simulink model "adcddcxaui"  (Simulink 8.1)
settings: Solver=ode45  StartTime=0.0  StopTime=100  RelTol=1e-3
libraries: xbsIndex_r4 x407, xbsIndex_r3 x127, xps_library x29, casper_library x5, casper_library_misc x4, casper_library_scopes x3
(part 1 of 6)
settings Model: Creator=andrew  LastModifiedBy=andrew
settings OptimizationCC: ExpressionDepthLimit=128  InitFltsAndDblsToZero=on
settings DebuggingCC: SaveWithParameterizedLinksMsg=none  SignalResolutionControl=TryResolveAllWithWarning  MultiTaskDSMMsg=warning  MultiTaskCondExecSysMsg=none  StrictBusMsg=None
settings RTWCC: IncludeERTFirstTime=on
settings GRTTargetCC: TargetFcnLib=ansi_tfl_tmw.mat

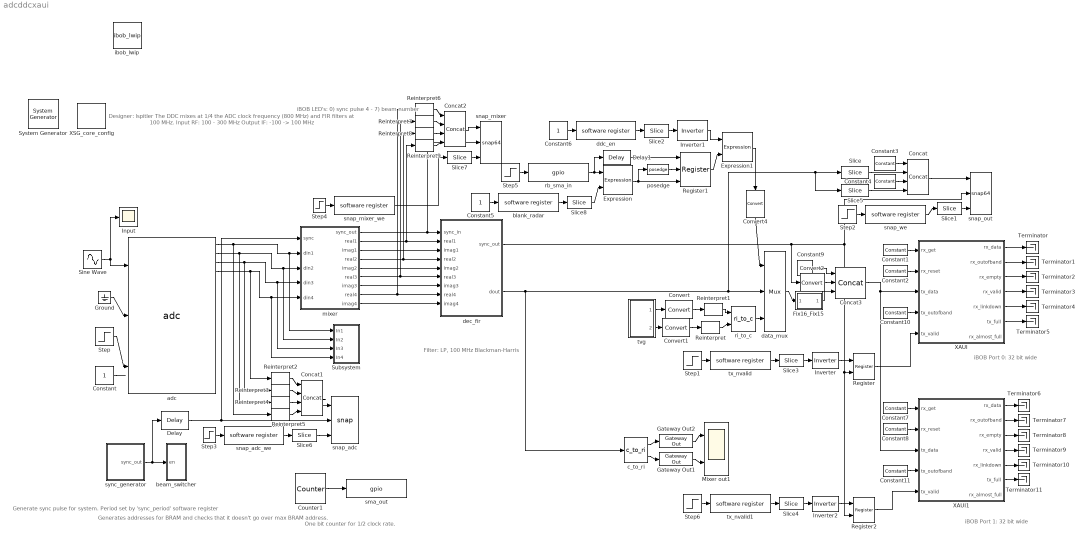
== system adcddcxaui ==
  note: Designer: lspitler
      | The DDC mixes at 1/4 the ADC clock frequency (800 MHz)
      | and FIR filters at 100 MHz.
      | Input RF: 100 - 300 MHz
      | Output IF: -100 -> 100 MHz
  note: Filter:
      | LP, 100 MHz Blackman-Harris
  note: iBOB Port 0: 32 bit wide
  note: One bit counter
      | for 1/2 clock rate.
  note: Generate sync pulse for system.
      | Period set by 'sync_period'
      | software register
  note: iBOB LED's:
      | 0) sync pulse
      | 4 - 7) beam number
  note: Generates addresses
      | for BRAM and checks
      | that it doesn't go over
      | max BRAM address.
  note: iBOB Port 1: 32 bit wide
  " System Generator" : xbsIndex_r4/ System Generator  Tag=genX  xilinxfamily=Kintex7  part=xc7k325t  speed=-3  package=fbg676  synthesis_tool=XST  clock_wrapper=Clock Enables  directory=./netlist  proj_type=Project Navigator  Synth_file=XST Defaults  Impl_file=ISE Defaults  testbench=off  simulink_period=1  sysclk_period=10  dcm_input_clock_period=10  incr_netlist=off  trim_vbits=Everywhere in SubSystem  dbl_ovrd=According to Block Masks  core_generation=According to Block Masks  run_coregen=off  deprecated_control=off  eval_field=0  block_type=sysgen
  Concat : xbsIndex_r3/Concat  num_inputs=4  explicit_period=on  period=1  dbl_ovrd=off
  Concat1 : xbsIndex_r3/Concat  num_inputs=4  explicit_period=on  period=1  dbl_ovrd=off
  Concat2 : xbsIndex_r3/Concat  num_inputs=4  explicit_period=on  period=1  dbl_ovrd=off
  Concat3 : xbsIndex_r3/Concat  num_inputs=3  explicit_period=on  period=1  dbl_ovrd=off
  Constant : Constant
  Constant1 : xbsIndex_r3/Constant  const=1  equ=P=C  arith_type=Boolean  n_bits=1  bin_pt=0  opselect=C  inp2=PCIN>>17  opr=+  inp1=P  carry=CIN  iostate=0  explicit_period=on  period=1  dbl_ovrd=off
  Constant10 : xbsIndex_r3/Constant  const=0  equ=P=C  arith_type=Unsigned  n_bits=4  bin_pt=0  opselect=C  inp2=PCIN>>17  opr=+  inp1=P  carry=CIN  iostate=0  explicit_period=on  period=1  dbl_ovrd=off
  Constant11 : xbsIndex_r3/Constant  const=0  equ=P=C  arith_type=Unsigned  n_bits=4  bin_pt=0  opselect=C  inp2=PCIN>>17  opr=+  inp1=P  carry=CIN  iostate=0  explicit_period=on  period=1  dbl_ovrd=off
  Constant2 : xbsIndex_r3/Constant  const=0  equ=P=C  arith_type=Boolean  n_bits=1  bin_pt=0  opselect=C  inp2=PCIN>>17  opr=+  inp1=P  carry=CIN  iostate=0  explicit_period=on  period=1  dbl_ovrd=off
  Constant3 : xbsIndex_r3/Constant  const=0  equ=P=C  arith_type=Unsigned  n_bits=16  bin_pt=0  opselect=C  inp2=PCIN>>17  opr=+  inp1=P  carry=CIN  iostate=0  explicit_period=on  period=1  dbl_ovrd=off
  Constant4 : xbsIndex_r3/Constant  const=0  equ=P=C  arith_type=Unsigned  n_bits=16  bin_pt=0  opselect=C  inp2=PCIN>>17  opr=+  inp1=P  carry=CIN  iostate=0  explicit_period=on  period=1  dbl_ovrd=off
  Constant5 : Constant
  Constant6 : Constant
  Constant7 : xbsIndex_r3/Constant  const=1  equ=P=C  arith_type=Boolean  n_bits=1  bin_pt=0  opselect=C  inp2=PCIN>>17  opr=+  inp1=P  carry=CIN  iostate=0  explicit_period=on  period=1  dbl_ovrd=off
  Constant8 : xbsIndex_r3/Constant  const=0  equ=P=C  arith_type=Boolean  n_bits=1  bin_pt=0  opselect=C  inp2=PCIN>>17  opr=+  inp1=P  carry=CIN  iostate=0  explicit_period=on  period=1  dbl_ovrd=off
  Constant9 : xbsIndex_r3/Constant  const=0  equ=P=C  arith_type=Unsigned  n_bits=1  bin_pt=0  opselect=C  inp2=PCIN>>17  opr=+  inp1=P  carry=CIN  iostate=0  explicit_period=on  period=1  dbl_ovrd=off
  Convert : xbsIndex_r3/Convert  arith_type=Unsigned  n_bits=16  bin_pt=0  quantization=Truncate  overflow=Wrap  latency=0  explicit_period=on  period=1  dbl_ovrd=off  show_param=off  inserted_by_tool=off  pipeline=off
      settings: xl_area=[0, 0, 0, 0, 0, 0, 0]
  Convert1 : xbsIndex_r3/Convert  arith_type=Unsigned  n_bits=16  bin_pt=0  quantization=Truncate  overflow=Wrap  latency=0  explicit_period=on  period=1  dbl_ovrd=off  show_param=off  inserted_by_tool=off  pipeline=off
      settings: xl_area=[0, 0, 0, 0, 0, 0, 0]
  Convert2 : xbsIndex_r3/Convert  arith_type=Unsigned  n_bits=1  bin_pt=0  quantization=Truncate  overflow=Wrap  latency=1  explicit_period=on  period=1  dbl_ovrd=off  show_param=off  inserted_by_tool=off  pipeline=off
      settings: xl_area=[0, 0, 0, 0, 0, 0, 0]
  Convert4 : xbsIndex_r3/Convert  arith_type=Unsigned  n_bits=1  bin_pt=0  quantization=Truncate  overflow=Wrap  latency=0  explicit_period=on  period=1  dbl_ovrd=off  show_param=off  inserted_by_tool=off  pipeline=off
      settings: xl_area=[0, 0, 0, 0, 0, 0, 0]
  Counter1 : xbsIndex_r3/Counter  cnt_type=Free Running  n_bits=1  bin_pt=0  arith_type=Unsigned  start_count=0  cnt_to=Inf  cnt_by_val=1  operation=Up  explicit_period=off  period=1  load_pin=off  rst=off  en=off  dbl_ovrd=off  show_param=off  use_rpm=on  gen_core=off
      settings: xl_area=[0, 0, 0, 0, 0, 0, 0]
  Delay : xbsIndex_r3/Delay  latency=8  reg_retiming=off  explicit_period=on  period=1  en=off  accept_only_valid=off  init_zero=on  dbl_ovrd=off  show_param=off
      settings: xl_area=[0, 0, 0, 0, 0, 0, 0]
  Delay1 : xbsIndex_r3/Delay  latency=1  reg_retiming=off  explicit_period=on  period=1  en=off  accept_only_valid=off  init_zero=on  dbl_ovrd=off  show_param=off
      settings: xl_area=[0, 0, 0, 0, 0, 0, 0]
  Expression : xbsIndex_r3/Expression  expression=a & b  precision=Full  arith_type=Unsigned  n_bits=8  bin_pt=2  align_bp=on  latency=1  explicit_period=on  period=1  en=off  dbl_ovrd=off  show_param=off
      settings: xl_area=[0, 0, 0, 0, 0, 0, 0]
  Expression1 : xbsIndex_r3/Expression  expression=a | b  precision=Full  arith_type=Unsigned  n_bits=8  bin_pt=2  align_bp=on  latency=0  explicit_period=on  period=1  en=off  dbl_ovrd=off  show_param=off
      settings: xl_area=[0, 0, 0, 0, 0, 0, 0]
  Fix16_Fix15 : Subsystem
  Gateway Out1 : xbsIndex_r3/Gateway Out  output_type=Double  nbits=8  bin_pt=6  arith_type=Boolean  quantization=Truncate  overflow=Wrap  hdl_port=on  timing_constraint=None  locs_specified=off  LOCs={}  needs_fixed_name=off  show_param=off
      settings: xl_area=[0, 0, 0, 0, 0, 0, 0]
  Gateway Out2 : xbsIndex_r3/Gateway Out  output_type=Double  nbits=8  bin_pt=6  arith_type=Boolean  quantization=Truncate  overflow=Wrap  hdl_port=on  timing_constraint=None  locs_specified=off  LOCs={}  needs_fixed_name=off  show_param=off
      settings: xl_area=[0, 0, 0, 0, 0, 0, 0]
  Ground : Ground
  Input : Scope
      settings: SaveName=ScopeData2
  Inverter : xbsIndex_r3/Inverter  latency=0  explicit_period=on  period=1  en=off  dbl_ovrd=off  show_param=off
      settings: xl_area=[0, 0, 0, 0, 0, 0, 0]
  Inverter1 : xbsIndex_r3/Inverter  latency=0  explicit_period=off  period=1  en=off  dbl_ovrd=off  show_param=off
      settings: xl_area=[0, 0, 0, 0, 0, 0, 0]
  Inverter2 : xbsIndex_r3/Inverter  latency=0  explicit_period=on  period=1  en=off  dbl_ovrd=off  show_param=off
      settings: xl_area=[0, 0, 0, 0, 0, 0, 0]
  Mixer out1 : Scope  NumInputPorts=2
      settings: YMin=-5~-5  YMax=5~5
  Register : xbsIndex_r3/Register  init=0  reg_only_valid=off  explicit_period=on  period=1  rst=off  en=on  out_en=off  dbl_ovrd=off  show_param=off
      settings: xl_area=[0, 0, 0, 0, 0, 0, 0]
  Register1 : xbsIndex_r3/Register  init=0  reg_only_valid=off  explicit_period=on  period=1  rst=on  en=on  out_en=off  dbl_ovrd=off  show_param=off
      settings: xl_area=[0, 0, 0, 0, 0, 0, 0]
  Register2 : xbsIndex_r3/Register  init=0  reg_only_valid=off  explicit_period=on  period=1  rst=off  en=on  out_en=off  dbl_ovrd=off  show_param=off
      settings: xl_area=[0, 0, 0, 0, 0, 0, 0]
  Reinterpret : xbsIndex_r3/Reinterpret  force_arith_type=on  arith_type="Signed  (2's comp)"  force_bin_pt=on  bin_pt=15  force_valid=on
  Reinterpret1 : xbsIndex_r3/Reinterpret  force_arith_type=on  arith_type="Signed  (2's comp)"  force_bin_pt=on  bin_pt=15  force_valid=on
  Reinterpret{2..9} (8 alike) : xbsIndex_r3/Reinterpret  force_arith_type=on  arith_type=Unsigned  force_bin_pt=on  bin_pt=0  force_valid=on
  Sine Wave : Sin  Amplitude=0.95  Frequency=2*3.1415*(11/8)  Samples=4  SampleTime=0.25  Offset=1
  Slice : xbsIndex_r3/Slice  mode=Upper Bit Location + Width  nbits=16  bit1=0  base1=MSB of Input  bit0=0  base0=LSB of Input  boolean_output=off  explicit_period=on  period=1  dbl_ovrd=off
  Slice{1..4,6..8} (7 alike) : xbsIndex_r3/Slice  mode=Lower Bit Location + Width  nbits=1  bit1=0  base1=MSB of Input  bit0=0  base0=LSB of Input  boolean_output=on  explicit_period=off  period=1  dbl_ovrd=off
  Slice5 : xbsIndex_r3/Slice  mode=Lower Bit Location + Width  nbits=16  bit1=0  base1=MSB of Input  bit0=0  base0=LSB of Input  boolean_output=off  explicit_period=on  period=1  dbl_ovrd=off
  Step{,1..6} (7 alike) : Step  SampleTime=0
  Subsystem : Subsystem
  Terminator{,1..11} (12 alike) : Terminator
  XAUI : Subsystem  Tag=xps:xaui  AncestorBlock=xps_library/XAUI  mask(xaui){demux=2, port=iBOB:0, show_param=off, pre_emph=3, swing=800}
      mask prompts: show_param "---------------------- Show Implementation Parameters -----------------------------------------------------------------------------------"; pre_emph "Pre-emphasis"; swing "Differential swing"
      mask help: XAUI block for sending and receiving point-to-point, streaming data over the BEE2 and iBOB's CX4 connectors. NOTE: A new version of this block is in development.
      mask init:
      | xaui_mask;
      mask Help: eval('xlWeb([getenv(''MLIB_ROOT''), ''\doc\html\com_xaui\com_xaui.html''])')
      mask TypeOptions demux: 1 | 2
      mask TypeOptions port: iBOB:0 | iBOB:1 | BEE2_ctrl:0 | BEE2_ctrl:1 | BEE2_usr:0 | BEE2_usr:1 | BEE2_usr:2 | BEE2_usr:3 | CORR:0
      mask Callback show_param:
      | myname=gcb;
      | if strcmp(get_param(myname, 'show_param'), 'on')
      |     set_param(myname, 'MaskVisibilities', {'on','on','on','on','on'});
      | else
      |     set_param(myname, 'MaskVisibilities', {'on','on','on','off','off'});
      | end
      mask TypeOptions pre_emph: 0 | 1 | 2 | 3
      mask TypeOptions swing: 400 | 500 | 600 | 700 | 800
  XAUI1 : Subsystem  Tag=xps:xaui  AncestorBlock=xps_library/XAUI  mask(xaui){demux=2, port=iBOB:1, show_param=off, pre_emph=3, swing=800}
      mask prompts: show_param "---------------------- Show Implementation Parameters -----------------------------------------------------------------------------------"; pre_emph "Pre-emphasis"; swing "Differential swing"
      mask help: XAUI block for sending and receiving point-to-point, streaming data over the BEE2 and iBOB's CX4 connectors. NOTE: A new version of this block is in development.
      mask init:
      | xaui_mask;
      mask Help: eval('xlWeb([getenv(''MLIB_ROOT''), ''\doc\html\com_xaui\com_xaui.html''])')
      mask TypeOptions demux: 1 | 2
      mask TypeOptions port: iBOB:0 | iBOB:1 | BEE2_ctrl:0 | BEE2_ctrl:1 | BEE2_usr:0 | BEE2_usr:1 | BEE2_usr:2 | BEE2_usr:3 | CORR:0
      mask Callback show_param:
      | myname=gcb;
      | if strcmp(get_param(myname, 'show_param'), 'on')
      |     set_param(myname, 'MaskVisibilities', {'on','on','on','on','on'});
      | else
      |     set_param(myname, 'MaskVisibilities', {'on','on','on','off','off'});
      | end
      mask TypeOptions pre_emph: 0 | 1 | 2 | 3
      mask TypeOptions swing: 400 | 500 | 600 | 700 | 800
  XSG_core_config : xps_library/XSG_core_config  Tag=xps:xsg  hw_sys=ROACH:sx95t  clk_src=sys_clk  ROACH_clk_src=sys_clk  ROACH2_clk_src=sys_clk  MKDIG_clk_src=sys_clk  clk_rate=100  sample_period=1  synthesis_tool=XST
  adc : xps_library/adc  Tag=xps:adc  adc_brd=adc0  adc_clk_rate=800  adc_interleave=off  sample_period=1
  beam_switcher : Subsystem
  blank_radar : xps_library/software register  Tag=xps:sw_reg  io_dir=From Processor  arith_type=Unsigned  bitwidth=32  bin_pt=0  sample_period=1  gw_name=adcddcxaui_blank_radar_user_data_out
  c_to_ri : casper_library_misc/c_to_ri  n_bits=16  bin_pt=15
      settings: AttributesFormatString=16_15 r/i
  data_mux : xbsIndex_r3/Mux  inputs=2  precision=Full  arith_type="Signed  (2's comp)"  n_bits=8  bin_pt=2  quantization=Truncate  overflow=Wrap  latency=2  explicit_period=on  period=1  en=off  dbl_ovrd=off  show_param=off  mux_type=off  use_rpm=off  gen_core=off
      settings: xl_area=[0, 0, 0, 0, 0, 0, 0]
  ddc_en : xps_library/software register  Tag=xps:sw_reg  io_dir=From Processor  arith_type=Unsigned  bitwidth=32  bin_pt=0  sample_period=1  gw_name=adcddcxaui_ddc_en_user_data_out
  dec_fir : Subsystem  AncestorBlock=casper_library/Downconverter/dec_fir  mask(dec_fir){n_inputs=4, coeff=getfield( getfield( get_param( gcb,'UserData'), 'parameters'),'coeff'), n_bits=16, quantization=Truncate, add_latency=2, mult_latency=2}
      mask prompts: n_inputs "Number of Parallel Streams"; coeff "Coefficients"; n_bits "Bit Width Out"; quantization "Quantization Behavior"; add_latency "Add Latency"; mult_latency "Mult Latency"
      mask help: FIR filter which can handle multiple time samples in parallel and decimates down to 1 time sample. If coefficients are symmetric, will automatically fold before multiplying.
      mask init:
      | dec_fir_init(gcb, ...
      |     'n_inputs', n_inputs, ...
      |     'coeff', coeff, ...
      |     'n_bits', n_bits, ...
      |     'quantization', quantization, ...
      |     'add_latency', add_latency, ...
      |     'mult_latency', mult_latency);
      settings: AttributesFormatString=|
      | 64 taps
      | 16_15 r/i
      mask Help:
      | <h1>Description</h1>
      | 
      | FIR filter which can handle multiple time samples in parallel and decimates down to 1 time sample.  If coefficients are symmetric, will automatically fold before multiplying.
      | 
      | <h2>Mask Parameters</h2>
      | 
      | <b>Number of Parallel Streams</b> (n_inputs): The number of time samples which arrive in parallel.<br><br>
      | 
      | <b>Coefficients</b> (coeff): The FIR coefficients.  If this vector is symmetric, the FIR will automatically fold before multiplying.<br><br>
      | 
      | <b>Bit Width Out</b> (n_bits): The number of bits in each real/imag sample of the complex number that is output.<br><br>
      | 
      | <b>Quantization Behavior</b> (quantization): The quantization behavior used in converting to the output bit width.<br><br>
      | 
      | 
      | <b>Add Latency</b> (add_latency) = The latency of adders/converters.<br><br>
      | 
      | <b>Mult Latency</b> (mult_latency) = The latency of multipliers.<br><br>
      mask TypeOptions quantization: Truncate | Round  (unbiased: +/- Inf) | Round  (unbiased: Even Values)
  ibob_lwip : xps_library/ibob_lwip
  mixer : Subsystem  AncestorBlock=casper_library/Downconverter/mixer  mask(mixer){freq_div=4, freq=1, nstreams=4, n_bits=8, bram_latency=2, mult_latency=3}
      mask prompts: freq_div "Frequency Divisions (M)"; freq "Mixing Frequency (? / M*2pi)"; nstreams "Number of Parallel Streams"; n_bits "Bit Width"; bram_latency "BRAM Latency"; mult_latency "Mult Latency"
      mask help: Digitally mixes an input signal (which can be several samples in parallel) with an LO of the indicated frequency (which is some fraction of the native FPGA clock rate).
      mask init:
      | mixer_init(gcb, ...
      |     'freq_div', freq_div, ...
      |     'freq', freq, ...
      |     'nstreams', nstreams, ...
      |     'n_bits', n_bits, ...
      |     'bram_latency', bram_latency, ...
      |     'mult_latency', mult_latency);
      settings: AttributesFormatString=lo at -1/4
      mask Help:
      | <h1>Description</h1>
      | 
      | Digitally mixes an input signal (which can be several samples in parallel) with an LO of the indicated frequency (which is some fraction of the native FPGA clock rate).
      | 
      | <h2>Mask Parameters</h2>
      | 
      | <b>Frequency Divisions</b> (freq_div):  The (power of 2) denominator of the mixing frequency. <br><br>
      | 
      | <b>Mixing Frequency</b> (freq) = The numerator of the mixing frequency.<br><br>
      | 
      | <b>Number of Parallel Streams</b> (nstreams) = The number of samples which arrive in parallel.<br><br>
      | 
      | <b>Bit Width</b> (n_bits) = The bitwidth of LO samples.<br><br>
      | 
      | <b>BRAM Latency</b> (bram_latency) = The latency of sine/cos lookup table.<br><br>
      | 
      | <b>MULT Latency</b> (mult_latency) = The latency of mixing multipliers.<br><br>
      | 
      | <h2> Usage </h2>
      | M = Frequency Divisions<br>
      | F = Mixing Frequency<br>
      | M and F must both be integers, and M must be a power of 2. The ratio F/M should equal the ratio f/r where r is the data rate of the sampled signal. For example, an F/M of 3/16 would downmix an 800Msps signal with an LO of 150MHz.
  posedge : casper_library_misc/posedge  Tag=Rising Edge Detector
  rb_sma_in : xps_library/gpio  Tag=xps:gpio  io_group=ROACH:aux0_clk  io_dir=in  arith_type=Boolean  bitwidth=1  bin_pt=0  bit_index=1  sample_period=1  use_single_ended=off  use_ddr=off  reg_iob=on  reg_clk_phase=0  termination=None
  ri_to_c : casper_library_misc/ri_to_c
  sma_out : xps_library/gpio  Tag=xps:gpio  io_group=ROACH:aux0_clk  io_dir=out  arith_type=Boolean  bitwidth=1  bin_pt=0  bit_index=0  sample_period=1  use_single_ended=off  use_ddr=off  reg_iob=on  reg_clk_phase=0  termination=None
  snap_adc : casper_library_scopes/snap  nsamples=11
  snap_adc_we : xps_library/software register  Tag=xps:sw_reg  io_dir=From Processor  arith_type=Unsigned  bitwidth=32  bin_pt=0  sample_period=1  gw_name=adcddcxaui_snap_adc_we_user_data_out
  snap_mixer : casper_library_scopes/snap64  nsamples=11
  snap_mixer_we : xps_library/software register  Tag=xps:sw_reg  io_dir=From Processor  arith_type=Unsigned  bitwidth=32  bin_pt=0  sample_period=1  gw_name=adcddcxaui_snap_mixer_we_user_data_out
  snap_out : casper_library_scopes/snap64  nsamples=11
  snap_we : xps_library/software register  Tag=xps:sw_reg  io_dir=From Processor  arith_type=Unsigned  bitwidth=32  bin_pt=0  sample_period=1  gw_name=adcddcxaui_snap_we_user_data_out
  sync_generator : Subsystem
  tvg : Subsystem
  tx_nvalid : xps_library/software register  Tag=xps:sw_reg  io_dir=From Processor  arith_type=Unsigned  bitwidth=32  bin_pt=0  sample_period=1  gw_name=adcddcxaui_tx_nvalid_user_data_out
  tx_nvalid1 : xps_library/software register  Tag=xps:sw_reg  io_dir=From Processor  arith_type=Unsigned  bitwidth=32  bin_pt=0  sample_period=1  gw_name=adcddcxaui_tx_nvalid1_user_data_out
  wires:
  mixer/1(sync_out) -> dec_fir/1(sync_in), snap_mixer/2
  mixer/2(real1) -> dec_fir/2(real1), Reinterpret9/1
  mixer/3(imag1) -> dec_fir/3(imag1)
  mixer/4(real2) -> dec_fir/4(real2), Reinterpret8/1
  mixer/5(imag2) -> dec_fir/5(imag2)
  mixer/6(real3) -> dec_fir/6(real3), Reinterpret7/1
  mixer/7(imag3) -> dec_fir/7(imag3)
  mixer/8(real4) -> dec_fir/8(real4), Reinterpret6/1
  mixer/9(imag4) -> dec_fir/9(imag4)
  dec_fir/2(dout) -> data_mux/2, Slice/1, Slice5/1, c_to_ri/1
  Constant1/1 -> XAUI/1(rx_get)
  Sine Wave/1 -> adc/1, Input/1
  Ground/1 -> adc/2
  adc/1 -> mixer/2(din1), Subsystem/1(In1), Reinterpret5/1
  adc/2 -> mixer/3(din2), Subsystem/2(In2), Reinterpret4/1
  adc/3 -> mixer/4(din3), Subsystem/3(In3), Reinterpret3/1
  adc/4 -> mixer/5(din4), Subsystem/4(In4), Reinterpret2/1
  Step/1 -> adc/3
  Constant/1 -> ?
  dec_fir/1(sync_out) -> snap_out/2, Register/2, Register2/2, Convert2/1
  snap_we/1 -> Slice1/1
  Step2/1 -> snap_we/1
  Slice1/1 -> snap_out/3
  XAUI/1(rx_data) -> Terminator/1
  XAUI/2(rx_outofband) -> Terminator1/1
  XAUI/3(rx_empty) -> Terminator2/1
  XAUI/4(rx_valid) -> Terminator3/1
  XAUI/5(rx_linkdown) -> Terminator4/1
  XAUI/6(tx_full) -> Terminator5/1
  Step1/1 -> tx_nvalid/1
  tx_nvalid/1 -> Slice3/1
  Inverter/1 -> Register/1
  Slice3/1 -> Inverter/1
  Register/1 -> XAUI/5(tx_valid)
  Expression1/1 -> Convert4/1
  tvg/1(re_out) -> Convert/1
  tvg/2(im_out) -> Convert1/1
  Convert/1 -> Reinterpret1/1
  Convert1/1 -> Reinterpret/1
  ri_to_c/1 -> data_mux/3
  Reinterpret1/1 -> ri_to_c/1
  Reinterpret/1 -> ri_to_c/2
  Counter1/1 -> sma_out/1
  sync_generator/1(sync_out) -> beam_switcher/1(en), Delay/1
  Delay/1 -> snap_adc/2, mixer/1(sync)
  Concat/1 -> snap_out/1
  Constant3/1 -> Concat/1
  Slice/1 -> Concat/2
  Constant4/1 -> Concat/3
  Slice5/1 -> Concat/4
  Reinterpret2/1 -> Concat1/1
  snap_adc_we/1 -> Slice6/1
  Step3/1 -> snap_adc_we/1
  Slice6/1 -> snap_adc/3
  Concat1/1 -> snap_adc/1
  Reinterpret3/1 -> Concat1/2
  Reinterpret4/1 -> Concat1/3
  Reinterpret5/1 -> Concat1/4
  snap_mixer_we/1 -> Slice7/1
  Step4/1 -> snap_mixer_we/1
  Slice7/1 -> snap_mixer/3
  Reinterpret6/1 -> Concat2/1
  Reinterpret7/1 -> Concat2/2
  Reinterpret8/1 -> Concat2/3
  Reinterpret9/1 -> Concat2/4
  Concat2/1 -> snap_mixer/1
  c_to_ri/2 -> Gateway Out1/1
  Gateway Out1/1 -> Mixer out1/2
  c_to_ri/1 -> Gateway Out2/1
  Gateway Out2/1 -> Mixer out1/1
  rb_sma_in/1 -> Expression/1, Delay1/1
  blank_radar/1 -> Slice8/1
  Slice8/1 -> Expression/2
  Constant5/1 -> blank_radar/1
  Step5/1 -> rb_sma_in/1
  Expression/1 -> Register1/3, posedge/1
  posedge/1 -> Register1/2
  Register1/1 -> Expression1/2
  Constant6/1 -> ddc_en/1
  ddc_en/1 -> Slice2/1
  Inverter1/1 -> Expression1/1
  Delay1/1 -> Register1/1
  Constant2/1 -> XAUI/2(rx_reset)
  Slice2/1 -> Inverter1/1
  Constant7/1 -> XAUI1/1(rx_get)
  Constant8/1 -> XAUI1/2(rx_reset)
  Step6/1 -> tx_nvalid1/1
  tx_nvalid1/1 -> Slice4/1
  Inverter2/1 -> Register2/1
  Slice4/1 -> Inverter2/1
  Register2/1 -> XAUI1/5(tx_valid)
  XAUI1/1(rx_data) -> Terminator6/1
  XAUI1/2(rx_outofband) -> Terminator7/1
  XAUI1/3(rx_empty) -> Terminator8/1
  XAUI1/4(rx_valid) -> Terminator9/1
  XAUI1/5(rx_linkdown) -> Terminator10/1
  XAUI1/6(tx_full) -> Terminator11/1
  Convert4/1 -> data_mux/1
  data_mux/1 -> Fix16_Fix15/1(In1)
  Constant9/1 -> Concat3/1
  Concat3/1 -> XAUI/3(tx_data), XAUI1/3(tx_data)
  Constant10/1 -> XAUI/4(tx_outofband)
  Constant11/1 -> XAUI1/4(tx_outofband)
  Fix16_Fix15/1(Out1) -> Concat3/3
  Convert2/1 -> Concat3/2

== system adcddcxaui/Fix16_Fix15 ==
  In1 : Inport
  Convert5 : xbsIndex_r3/Convert  arith_type="Signed  (2's comp)"  n_bits=15  bin_pt=14  quantization=Truncate  overflow=Wrap  latency=0  explicit_period=on  period=1  dbl_ovrd=off  show_param=off  inserted_by_tool=off  pipeline=off
      settings: xl_area=[0, 0, 0, 0, 0, 0, 0]
  Convert6 : xbsIndex_r3/Convert  arith_type="Signed  (2's comp)"  n_bits=15  bin_pt=14  quantization=Truncate  overflow=Wrap  latency=0  explicit_period=on  period=1  dbl_ovrd=off  show_param=off  inserted_by_tool=off  pipeline=off
      settings: xl_area=[0, 0, 0, 0, 0, 0, 0]
  c_to_ri1 : casper_library/Misc/c_to_ri  n_bits=16  bin_pt=15
      settings: AttributesFormatString=16_15 r/i
  ri_to_c1 : casper_library/Misc/ri_to_c
  Out1 : Outport
  wires:
  c_to_ri1/1 -> Convert5/1
  c_to_ri1/2 -> Convert6/1
  Convert5/1 -> ri_to_c1/1
  Convert6/1 -> ri_to_c1/2
  In1/1 -> c_to_ri1/1
  ri_to_c1/1 -> Out1/1

== system adcddcxaui/Subsystem ==
  In1 : Inport
  In2 : Inport  Port=2
  In3 : Inport  Port=3
  In4 : Inport  Port=4
  ADC out : Scope  NumInputPorts=4
      settings: YMin=-5~-5~-5~-5  YMax=5~5~5~5  SaveName=ScopeData3
  Gateway Out{2..5} (4 alike) : xbsIndex_r3/Gateway Out  output_type=Double  nbits=8  bin_pt=6  arith_type=Boolean  quantization=Truncate  overflow=Wrap  hdl_port=on  timing_constraint=None  locs_specified=off  LOCs={}  needs_fixed_name=off  show_param=off
      settings: xl_area=[0, 0, 0, 0, 0, 0, 0]
  wires:
  Gateway Out2/1 -> ADC out/1
  Gateway Out3/1 -> ADC out/2
  Gateway Out4/1 -> ADC out/3
  Gateway Out5/1 -> ADC out/4
  In1/1 -> Gateway Out2/1
  In2/1 -> Gateway Out3/1
  In3/1 -> Gateway Out4/1
  In4/1 -> Gateway Out5/1

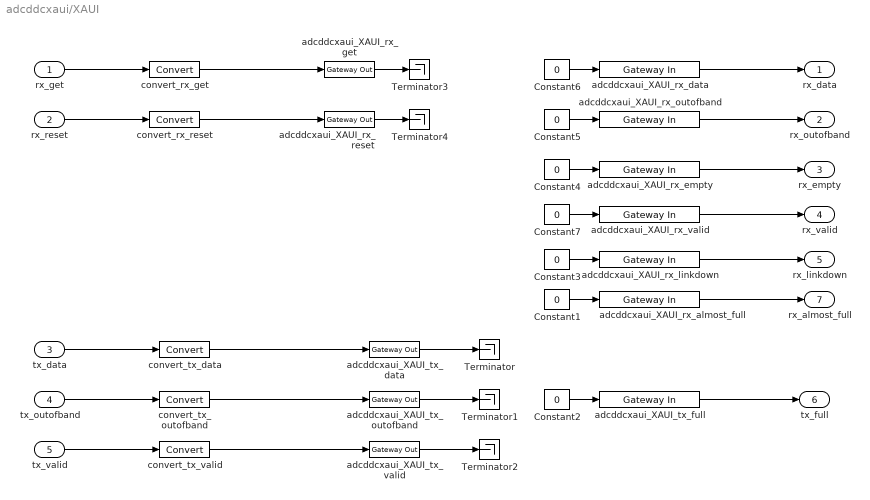
== system adcddcxaui/XAUI ==
  rx_get : Inport
  rx_reset : Inport  Port=2
  tx_data : Inport  Port=3
  tx_outofband : Inport  Port=4
  tx_valid : Inport  Port=5
  Constant{1..7} (7 alike) : Constant  Value=0
  Terminator{,1..4} (5 alike) : Terminator
  adcddcxaui_XAUI_rx_almost_full : xbsIndex_r3/Gateway In  arith_type=Boolean  n_bits=1  bin_pt=0  quantization=Truncate  overflow=Wrap  period=1  timing_constraint=None  locs_specified=off  LOCs={}  needs_fixed_name=off  dbl_ovrd=off  show_param=off
      settings: xl_area=[0, 0, 0, 0, 0, 0, 0]
  adcddcxaui_XAUI_rx_data : xbsIndex_r3/Gateway In  arith_type=Unsigned  n_bits=32  bin_pt=0  quantization=Truncate  overflow=Wrap  period=1  timing_constraint=None  locs_specified=off  LOCs={}  needs_fixed_name=off  dbl_ovrd=off  show_param=off
      settings: xl_area=[0, 0, 0, 0, 0, 0, 0]
  adcddcxaui_XAUI_rx_empty : xbsIndex_r3/Gateway In  arith_type=Boolean  n_bits=1  bin_pt=0  quantization=Truncate  overflow=Wrap  period=1  timing_constraint=None  locs_specified=off  LOCs={}  needs_fixed_name=off  dbl_ovrd=off  show_param=off
      settings: xl_area=[0, 0, 0, 0, 0, 0, 0]
  adcddcxaui_XAUI_rx_get : xbsIndex_r3/Gateway Out  output_type=Double  nbits=8  bin_pt=6  arith_type=Boolean  quantization=Truncate  overflow=Wrap  hdl_port=on  timing_constraint=None  locs_specified=off  LOCs={}  needs_fixed_name=off  show_param=off
      settings: xl_area=[0, 0, 0, 0, 0, 0, 0]
  adcddcxaui_XAUI_rx_linkdown : xbsIndex_r3/Gateway In  arith_type=Boolean  n_bits=1  bin_pt=0  quantization=Truncate  overflow=Wrap  period=1  timing_constraint=None  locs_specified=off  LOCs={}  needs_fixed_name=off  dbl_ovrd=off  show_param=off
      settings: xl_area=[0, 0, 0, 0, 0, 0, 0]
  adcddcxaui_XAUI_rx_outofband : xbsIndex_r3/Gateway In  arith_type=Unsigned  n_bits=4  bin_pt=0  quantization=Truncate  overflow=Wrap  period=1  timing_constraint=None  locs_specified=off  LOCs={}  needs_fixed_name=off  dbl_ovrd=off  show_param=off
      settings: xl_area=[0, 0, 0, 0, 0, 0, 0]
  adcddcxaui_XAUI_rx_reset : xbsIndex_r3/Gateway Out  output_type=Double  nbits=8  bin_pt=6  arith_type=Boolean  quantization=Truncate  overflow=Wrap  hdl_port=on  timing_constraint=None  locs_specified=off  LOCs={}  needs_fixed_name=off  show_param=off
      settings: xl_area=[0, 0, 0, 0, 0, 0, 0]
  adcddcxaui_XAUI_rx_valid : xbsIndex_r3/Gateway In  arith_type=Boolean  n_bits=1  bin_pt=0  quantization=Truncate  overflow=Wrap  period=1  timing_constraint=None  locs_specified=off  LOCs={}  needs_fixed_name=off  dbl_ovrd=off  show_param=off
      settings: xl_area=[0, 0, 0, 0, 0, 0, 0]
  adcddcxaui_XAUI_tx_data : xbsIndex_r3/Gateway Out  output_type=Double  nbits=8  bin_pt=6  arith_type=Boolean  quantization=Truncate  overflow=Wrap  hdl_port=on  timing_constraint=None  locs_specified=off  LOCs={}  needs_fixed_name=off  show_param=off
      settings: xl_area=[0, 0, 0, 0, 0, 0, 0]
  adcddcxaui_XAUI_tx_full : xbsIndex_r3/Gateway In  arith_type=Boolean  n_bits=1  bin_pt=0  quantization=Truncate  overflow=Wrap  period=1  timing_constraint=None  locs_specified=off  LOCs={}  needs_fixed_name=off  dbl_ovrd=off  show_param=off
      settings: xl_area=[0, 0, 0, 0, 0, 0, 0]
  adcddcxaui_XAUI_tx_outofband : xbsIndex_r3/Gateway Out  output_type=Double  nbits=8  bin_pt=6  arith_type=Boolean  quantization=Truncate  overflow=Wrap  hdl_port=on  timing_constraint=None  locs_specified=off  LOCs={}  needs_fixed_name=off  show_param=off
      settings: xl_area=[0, 0, 0, 0, 0, 0, 0]
  adcddcxaui_XAUI_tx_valid : xbsIndex_r3/Gateway Out  output_type=Double  nbits=8  bin_pt=6  arith_type=Boolean  quantization=Truncate  overflow=Wrap  hdl_port=on  timing_constraint=None  locs_specified=off  LOCs={}  needs_fixed_name=off  show_param=off
      settings: xl_area=[0, 0, 0, 0, 0, 0, 0]
  convert_rx_get : xbsIndex_r3/Convert  arith_type=Boolean  n_bits=64  bin_pt=0  quantization=Truncate  overflow=Wrap  latency=0  explicit_period=off  period=1  dbl_ovrd=off  show_param=off  inserted_by_tool=off  pipeline=off
      settings: xl_area=[0, 0, 0, 0, 0, 0, 0]
  convert_rx_reset : xbsIndex_r3/Convert  arith_type=Boolean  n_bits=1  bin_pt=0  quantization=Truncate  overflow=Wrap  latency=0  explicit_period=off  period=1  dbl_ovrd=off  show_param=off  inserted_by_tool=off  pipeline=off
      settings: xl_area=[0, 0, 0, 0, 0, 0, 0]
  convert_tx_data : xbsIndex_r3/Convert  arith_type=Unsigned  n_bits=32  bin_pt=0  quantization=Truncate  overflow=Wrap  latency=0  explicit_period=off  period=1  dbl_ovrd=off  show_param=off  inserted_by_tool=off  pipeline=off
      settings: xl_area=[0, 0, 0, 0, 0, 0, 0]
  convert_tx_outofband : xbsIndex_r3/Convert  arith_type=Unsigned  n_bits=4  bin_pt=0  quantization=Truncate  overflow=Wrap  latency=0  explicit_period=off  period=1  dbl_ovrd=off  show_param=off  inserted_by_tool=off  pipeline=off
      settings: xl_area=[0, 0, 0, 0, 0, 0, 0]
  convert_tx_valid : xbsIndex_r3/Convert  arith_type=Boolean  n_bits=1  bin_pt=0  quantization=Truncate  overflow=Wrap  latency=0  explicit_period=off  period=1  dbl_ovrd=off  show_param=off  inserted_by_tool=off  pipeline=off
      settings: xl_area=[0, 0, 0, 0, 0, 0, 0]
  rx_data : Outport
  rx_outofband : Outport  Port=2
  rx_empty : Outport  Port=3
  rx_valid : Outport  Port=4
  rx_linkdown : Outport  Port=5
  tx_full : Outport  Port=6
  rx_almost_full : Outport  Port=7
  wires:
  Constant1/1 -> adcddcxaui_XAUI_rx_almost_full/1
  adcddcxaui_XAUI_rx_almost_full/1 -> rx_almost_full/1
  adcddcxaui_XAUI_rx_valid/1 -> rx_valid/1
  Constant7/1 -> adcddcxaui_XAUI_rx_valid/1
  adcddcxaui_XAUI_rx_reset/1 -> Terminator4/1
  adcddcxaui_XAUI_rx_get/1 -> Terminator3/1
  Constant6/1 -> adcddcxaui_XAUI_rx_data/1
  Constant5/1 -> adcddcxaui_XAUI_rx_outofband/1
  Constant4/1 -> adcddcxaui_XAUI_rx_empty/1
  Constant3/1 -> adcddcxaui_XAUI_rx_linkdown/1
  Constant2/1 -> adcddcxaui_XAUI_tx_full/1
  adcddcxaui_XAUI_tx_valid/1 -> Terminator2/1
  adcddcxaui_XAUI_tx_outofband/1 -> Terminator1/1
  adcddcxaui_XAUI_tx_data/1 -> Terminator/1
  adcddcxaui_XAUI_tx_full/1 -> tx_full/1
  convert_tx_valid/1 -> adcddcxaui_XAUI_tx_valid/1
  tx_valid/1 -> convert_tx_valid/1
  convert_tx_outofband/1 -> adcddcxaui_XAUI_tx_outofband/1
  tx_outofband/1 -> convert_tx_outofband/1
  convert_tx_data/1 -> adcddcxaui_XAUI_tx_data/1
  tx_data/1 -> convert_tx_data/1
  adcddcxaui_XAUI_rx_linkdown/1 -> rx_linkdown/1
  adcddcxaui_XAUI_rx_empty/1 -> rx_empty/1
  adcddcxaui_XAUI_rx_outofband/1 -> rx_outofband/1
  adcddcxaui_XAUI_rx_data/1 -> rx_data/1
  convert_rx_reset/1 -> adcddcxaui_XAUI_rx_reset/1
  rx_reset/1 -> convert_rx_reset/1
  convert_rx_get/1 -> adcddcxaui_XAUI_rx_get/1
  rx_get/1 -> convert_rx_get/1

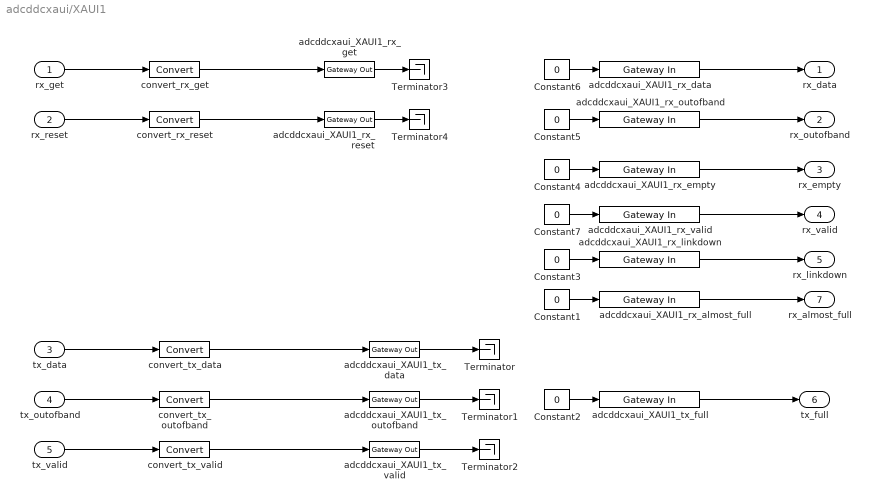
== system adcddcxaui/XAUI1 ==
  rx_get : Inport
  rx_reset : Inport  Port=2
  tx_data : Inport  Port=3
  tx_outofband : Inport  Port=4
  tx_valid : Inport  Port=5
  Constant{1..7} (7 alike) : Constant  Value=0
  Terminator{,1..4} (5 alike) : Terminator
  adcddcxaui_XAUI1_rx_almost_full : xbsIndex_r3/Gateway In  arith_type=Boolean  n_bits=1  bin_pt=0  quantization=Truncate  overflow=Wrap  period=1  timing_constraint=None  locs_specified=off  LOCs={}  needs_fixed_name=off  dbl_ovrd=off  show_param=off
      settings: xl_area=[0, 0, 0, 0, 0, 0, 0]
  adcddcxaui_XAUI1_rx_data : xbsIndex_r3/Gateway In  arith_type=Unsigned  n_bits=32  bin_pt=0  quantization=Truncate  overflow=Wrap  period=1  timing_constraint=None  locs_specified=off  LOCs={}  needs_fixed_name=off  dbl_ovrd=off  show_param=off
      settings: xl_area=[0, 0, 0, 0, 0, 0, 0]
  adcddcxaui_XAUI1_rx_empty : xbsIndex_r3/Gateway In  arith_type=Boolean  n_bits=1  bin_pt=0  quantization=Truncate  overflow=Wrap  period=1  timing_constraint=None  locs_specified=off  LOCs={}  needs_fixed_name=off  dbl_ovrd=off  show_param=off
      settings: xl_area=[0, 0, 0, 0, 0, 0, 0]
  adcddcxaui_XAUI1_rx_get : xbsIndex_r3/Gateway Out  output_type=Double  nbits=8  bin_pt=6  arith_type=Boolean  quantization=Truncate  overflow=Wrap  hdl_port=on  timing_constraint=None  locs_specified=off  LOCs={}  needs_fixed_name=off  show_param=off
      settings: xl_area=[0, 0, 0, 0, 0, 0, 0]
  adcddcxaui_XAUI1_rx_linkdown : xbsIndex_r3/Gateway In  arith_type=Boolean  n_bits=1  bin_pt=0  quantization=Truncate  overflow=Wrap  period=1  timing_constraint=None  locs_specified=off  LOCs={}  needs_fixed_name=off  dbl_ovrd=off  show_param=off
      settings: xl_area=[0, 0, 0, 0, 0, 0, 0]
  adcddcxaui_XAUI1_rx_outofband : xbsIndex_r3/Gateway In  arith_type=Unsigned  n_bits=4  bin_pt=0  quantization=Truncate  overflow=Wrap  period=1  timing_constraint=None  locs_specified=off  LOCs={}  needs_fixed_name=off  dbl_ovrd=off  show_param=off
      settings: xl_area=[0, 0, 0, 0, 0, 0, 0]
  adcddcxaui_XAUI1_rx_reset : xbsIndex_r3/Gateway Out  output_type=Double  nbits=8  bin_pt=6  arith_type=Boolean  quantization=Truncate  overflow=Wrap  hdl_port=on  timing_constraint=None  locs_specified=off  LOCs={}  needs_fixed_name=off  show_param=off
      settings: xl_area=[0, 0, 0, 0, 0, 0, 0]
  adcddcxaui_XAUI1_rx_valid : xbsIndex_r3/Gateway In  arith_type=Boolean  n_bits=1  bin_pt=0  quantization=Truncate  overflow=Wrap  period=1  timing_constraint=None  locs_specified=off  LOCs={}  needs_fixed_name=off  dbl_ovrd=off  show_param=off
      settings: xl_area=[0, 0, 0, 0, 0, 0, 0]
  adcddcxaui_XAUI1_tx_data : xbsIndex_r3/Gateway Out  output_type=Double  nbits=8  bin_pt=6  arith_type=Boolean  quantization=Truncate  overflow=Wrap  hdl_port=on  timing_constraint=None  locs_specified=off  LOCs={}  needs_fixed_name=off  show_param=off
      settings: xl_area=[0, 0, 0, 0, 0, 0, 0]
  adcddcxaui_XAUI1_tx_full : xbsIndex_r3/Gateway In  arith_type=Boolean  n_bits=1  bin_pt=0  quantization=Truncate  overflow=Wrap  period=1  timing_constraint=None  locs_specified=off  LOCs={}  needs_fixed_name=off  dbl_ovrd=off  show_param=off
      settings: xl_area=[0, 0, 0, 0, 0, 0, 0]
  adcddcxaui_XAUI1_tx_outofband : xbsIndex_r3/Gateway Out  output_type=Double  nbits=8  bin_pt=6  arith_type=Boolean  quantization=Truncate  overflow=Wrap  hdl_port=on  timing_constraint=None  locs_specified=off  LOCs={}  needs_fixed_name=off  show_param=off
      settings: xl_area=[0, 0, 0, 0, 0, 0, 0]
  adcddcxaui_XAUI1_tx_valid : xbsIndex_r3/Gateway Out  output_type=Double  nbits=8  bin_pt=6  arith_type=Boolean  quantization=Truncate  overflow=Wrap  hdl_port=on  timing_constraint=None  locs_specified=off  LOCs={}  needs_fixed_name=off  show_param=off
      settings: xl_area=[0, 0, 0, 0, 0, 0, 0]
  convert_rx_get : xbsIndex_r3/Convert  arith_type=Boolean  n_bits=64  bin_pt=0  quantization=Truncate  overflow=Wrap  latency=0  explicit_period=off  period=1  dbl_ovrd=off  show_param=off  inserted_by_tool=off  pipeline=off
      settings: xl_area=[0, 0, 0, 0, 0, 0, 0]
  convert_rx_reset : xbsIndex_r3/Convert  arith_type=Boolean  n_bits=1  bin_pt=0  quantization=Truncate  overflow=Wrap  latency=0  explicit_period=off  period=1  dbl_ovrd=off  show_param=off  inserted_by_tool=off  pipeline=off
      settings: xl_area=[0, 0, 0, 0, 0, 0, 0]
  convert_tx_data : xbsIndex_r3/Convert  arith_type=Unsigned  n_bits=32  bin_pt=0  quantization=Truncate  overflow=Wrap  latency=0  explicit_period=off  period=1  dbl_ovrd=off  show_param=off  inserted_by_tool=off  pipeline=off
      settings: xl_area=[0, 0, 0, 0, 0, 0, 0]
  convert_tx_outofband : xbsIndex_r3/Convert  arith_type=Unsigned  n_bits=4  bin_pt=0  quantization=Truncate  overflow=Wrap  latency=0  explicit_period=off  period=1  dbl_ovrd=off  show_param=off  inserted_by_tool=off  pipeline=off
      settings: xl_area=[0, 0, 0, 0, 0, 0, 0]
  convert_tx_valid : xbsIndex_r3/Convert  arith_type=Boolean  n_bits=1  bin_pt=0  quantization=Truncate  overflow=Wrap  latency=0  explicit_period=off  period=1  dbl_ovrd=off  show_param=off  inserted_by_tool=off  pipeline=off
      settings: xl_area=[0, 0, 0, 0, 0, 0, 0]
  rx_data : Outport
  rx_outofband : Outport  Port=2
  rx_empty : Outport  Port=3
  rx_valid : Outport  Port=4
  rx_linkdown : Outport  Port=5
  tx_full : Outport  Port=6
  rx_almost_full : Outport  Port=7
  wires:
  rx_get/1 -> convert_rx_get/1
  convert_rx_get/1 -> adcddcxaui_XAUI1_rx_get/1
  rx_reset/1 -> convert_rx_reset/1
  convert_rx_reset/1 -> adcddcxaui_XAUI1_rx_reset/1
  adcddcxaui_XAUI1_rx_data/1 -> rx_data/1
  adcddcxaui_XAUI1_rx_outofband/1 -> rx_outofband/1
  adcddcxaui_XAUI1_rx_empty/1 -> rx_empty/1
  adcddcxaui_XAUI1_rx_linkdown/1 -> rx_linkdown/1
  tx_data/1 -> convert_tx_data/1
  convert_tx_data/1 -> adcddcxaui_XAUI1_tx_data/1
  tx_outofband/1 -> convert_tx_outofband/1
  convert_tx_outofband/1 -> adcddcxaui_XAUI1_tx_outofband/1
  tx_valid/1 -> convert_tx_valid/1
  convert_tx_valid/1 -> adcddcxaui_XAUI1_tx_valid/1
  adcddcxaui_XAUI1_tx_full/1 -> tx_full/1
  adcddcxaui_XAUI1_tx_data/1 -> Terminator/1
  adcddcxaui_XAUI1_tx_outofband/1 -> Terminator1/1
  adcddcxaui_XAUI1_tx_valid/1 -> Terminator2/1
  Constant2/1 -> adcddcxaui_XAUI1_tx_full/1
  Constant3/1 -> adcddcxaui_XAUI1_rx_linkdown/1
  Constant4/1 -> adcddcxaui_XAUI1_rx_empty/1
  Constant5/1 -> adcddcxaui_XAUI1_rx_outofband/1
  Constant6/1 -> adcddcxaui_XAUI1_rx_data/1
  adcddcxaui_XAUI1_rx_get/1 -> Terminator3/1
  adcddcxaui_XAUI1_rx_reset/1 -> Terminator4/1
  Constant7/1 -> adcddcxaui_XAUI1_rx_valid/1
  adcddcxaui_XAUI1_rx_valid/1 -> rx_valid/1
  adcddcxaui_XAUI1_rx_almost_full/1 -> rx_almost_full/1
  Constant1/1 -> adcddcxaui_XAUI1_rx_almost_full/1

== system adcddcxaui/beam_switcher ==
  note: Generates addresses
      | in read mode.
      | 'en' comes from sync
      | pulse
  note: Latency through
      | system is about 3.
  en : Inport
  8 LSB : xbsIndex_r3/Slice  mode=Lower Bit Location + Width  nbits=8  bit1=10  base1=MSB of Input  bit0=0  base0=LSB of Input  boolean_output=off  explicit_period=on  period=1  dbl_ovrd=off
  8 LSB1 : xbsIndex_r3/Slice  mode=Lower Bit Location + Width  nbits=8  bit1=10  base1=MSB of Input  bit0=0  base0=LSB of Input  boolean_output=off  explicit_period=on  period=1  dbl_ovrd=off
  Constant : Constant
  Constant1 : xbsIndex_r3/Constant  const=0  equ=P=C  arith_type=Boolean  n_bits=32  bin_pt=0  opselect=C  inp2=PCIN>>17  opr=+  inp1=P  carry=CIN  iostate=0  explicit_period=on  period=1  dbl_ovrd=off
  Constant6 : xbsIndex_r3/Constant  const=0  equ=P=C  arith_type=Unsigned  n_bits=32  bin_pt=0  opselect=C  inp2=PCIN>>17  opr=+  inp1=P  carry=CIN  iostate=0  explicit_period=on  period=1  dbl_ovrd=off
  Counter2 : xbsIndex_r3/Counter  cnt_type=Free Running  n_bits=11  bin_pt=0  arith_type=Unsigned  start_count=0  cnt_to=Inf  cnt_by_val=1  operation=Up  explicit_period=on  period=1  load_pin=off  rst=on  en=on  dbl_ovrd=off  show_param=off  use_rpm=on  gen_core=off
      settings: xl_area=[0, 0, 0, 0, 0, 0, 0]
  Gateway Out12 : xbsIndex_r3/Gateway Out  output_type=Double  nbits=8  bin_pt=6  arith_type=Boolean  quantization=Truncate  overflow=Wrap  hdl_port=on  timing_constraint=None  locs_specified=off  LOCs={}  needs_fixed_name=off  show_param=off
      settings: xl_area=[0, 0, 0, 0, 0, 0, 0]
  Gateway Out13 : xbsIndex_r3/Gateway Out  output_type=Double  nbits=8  bin_pt=6  arith_type=Boolean  quantization=Truncate  overflow=Wrap  hdl_port=on  timing_constraint=None  locs_specified=off  LOCs={}  needs_fixed_name=off  show_param=off
      settings: xl_area=[0, 0, 0, 0, 0, 0, 0]
  Relational1 : xbsIndex_r3/Relational  mode=a>=b  latency=1  explicit_period=on  period=1  en=off  dbl_ovrd=off  show_param=off
      settings: xl_area=[0, 0, 0, 0, 0, 0, 0]
  beam switch : Scope  NumInputPorts=2
      settings: YMin=-5~-5  YMax=5~5  SaveName=ScopeData6
  beam_leds : Subsystem
  beam_number : xps_library/software register  Tag=xps:sw_reg  io_dir=To Processor  arith_type=Unsigned  bitwidth=32  bin_pt=0  sample_period=1  gw_name=adcddcxaui_beam_switcher_beam_number_user_data_in
  gpio0 : xps_library/gpio  Tag=xps:gpio  io_group=iBOB:gpio0  io_dir=out  arith_type=Unsigned  bitwidth=8  bin_pt=0  bit_index=[0:7]  sample_period=1  use_single_ended=off  use_ddr=off  reg_iob=on  reg_clk_phase=0  termination=None
  gpio3 : xps_library/gpio  Tag=xps:gpio  io_group=iBOB:gpio3  io_dir=out  arith_type=Unsigned  bitwidth=8  bin_pt=0  bit_index=[0:7]  sample_period=1  use_single_ended=off  use_ddr=off  reg_iob=on  reg_clk_phase=0  termination=None
  max_addr : xps_library/software register  Tag=xps:sw_reg  io_dir=From Processor  arith_type=Unsigned  bitwidth=32  bin_pt=0  sample_period=1  gw_name=adcddcxaui_beam_switcher_max_addr_user_data_out
  switchyard_BRAM : xps_library/Shared BRAM  Tag=xps:bram  arith_type=Unsigned  addr_width=11  data_width=32  data_bin_pt=0  init_vals=[0:2^11-1]  sample_rate=1
  wires:
  Counter2/1 -> Gateway Out12/1, switchyard_BRAM/1, Relational1/1
  Relational1/1 -> Counter2/1, Gateway Out13/1
  switchyard_BRAM/1 -> beam_number/1, beam_leds/1(In), 8 LSB/1, 8 LSB1/1
  en/1 -> Counter2/2
  Gateway Out12/1 -> beam switch/1
  Gateway Out13/1 -> beam switch/2
  Constant/1 -> max_addr/1
  8 LSB/1 -> gpio0/1
  8 LSB1/1 -> gpio3/1
  max_addr/1 -> Relational1/2
  Constant6/1 -> switchyard_BRAM/2
  Constant1/1 -> switchyard_BRAM/3
